simulink model "Overall_Mission"  (R2019b)
settings: Solver=VariableStepAuto  StartTime=0.0  StopTime=10.0  RelTol=1e-3
settings Model: Creator=visha  LastModifiedBy=visha
settings OptimizationCC: DefaultParameterBehavior=Inlined

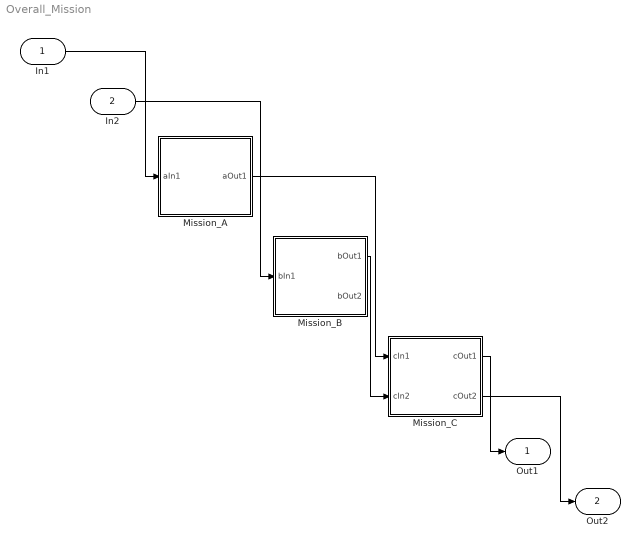
== system Overall_Mission ==
  In1 : Inport  OutDataTypeStr=double
  In2 : Inport  Port=2  OutDataTypeStr=int32
  Mission_A : Subsystem
  Mission_B : Subsystem
  Mission_C : Subsystem
  Out1 : Outport  OutDataTypeStr=double
  Out2 : Outport  Port=2  OutDataTypeStr=boolean
  wires:
  In1/1 -> Mission_A/1(aIn1)
  In2/1 -> Mission_B/1(bIn1)
  Mission_A/1(aOut1) -> Mission_C/1(cIn1)
  Mission_B/1(bOut1) -> Mission_C/2(cIn2)
  Mission_C/1(cOut1) -> Out1/1
  Mission_C/2(cOut2) -> Out2/1

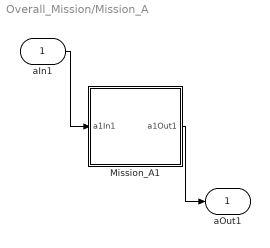
== system Overall_Mission/Mission_A ==
  aIn1 : Inport  OutDataTypeStr=double
  Mission_A1 : Subsystem
  aOut1 : Outport  OutDataTypeStr=double
  wires:
  Mission_A1/1(a1Out1) -> aOut1/1
  aIn1/1 -> Mission_A1/1(a1In1)

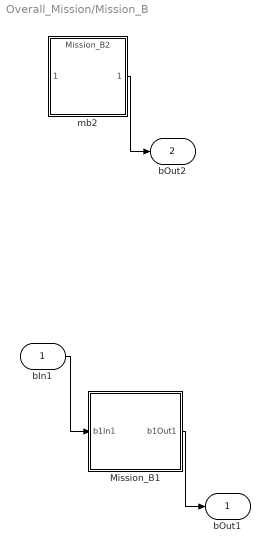
== system Overall_Mission/Mission_B ==
  bIn1 : Inport  OutDataTypeStr=int32
  Mission_B1 : Subsystem
  mb2 : ModelReference  ModelNameDialog=Mission_B2  SimulationMode=Normal  ModelReferenceVersion=1.1
  bOut1 : Outport  OutDataTypeStr=int32
  bOut2 : Outport  Port=2  OutDataTypeStr=int32
  wires:
  bIn1/1 -> Mission_B1/1(b1In1)
  Mission_B1/1(b1Out1) -> bOut1/1
  mb2/1 -> bOut2/1

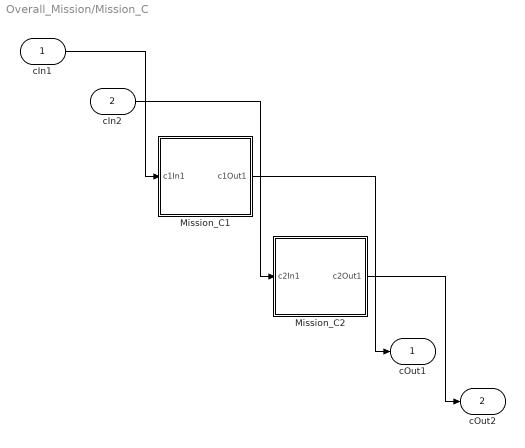
== system Overall_Mission/Mission_C ==
  cIn1 : Inport  OutDataTypeStr=double
  cIn2 : Inport  Port=2  OutDataTypeStr=int32
  Mission_C1 : Subsystem
  Mission_C2 : Subsystem
  cOut1 : Outport  OutDataTypeStr=double
  cOut2 : Outport  Port=2  OutDataTypeStr=boolean
  wires:
  cIn1/1 -> Mission_C1/1(c1In1)
  cIn2/1 -> Mission_C2/1(c2In1)
  Mission_C1/1(c1Out1) -> cOut1/1
  Mission_C2/1(c2Out1) -> cOut2/1

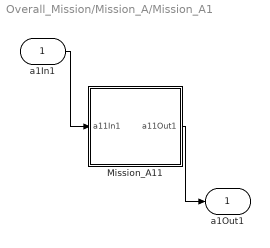
== system Overall_Mission/Mission_A/Mission_A1 ==
  a1In1 : Inport  OutDataTypeStr=double
  Mission_A11 : Subsystem
  a1Out1 : Outport  OutDataTypeStr=double
  wires:
  a1In1/1 -> Mission_A11/1(a11In1)
  Mission_A11/1(a11Out1) -> a1Out1/1

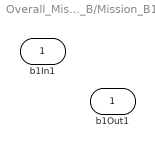
== system Overall_Mission/Mission_B/Mission_B1 ==
  b1In1 : Inport  OutDataTypeStr=int32
  b1Out1 : Outport  OutDataTypeStr=int32

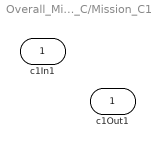
== system Overall_Mission/Mission_C/Mission_C1 ==
  c1In1 : Inport  OutDataTypeStr=double
  c1Out1 : Outport  OutDataTypeStr=double

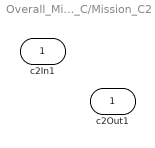
== system Overall_Mission/Mission_C/Mission_C2 ==
  c2In1 : Inport  OutDataTypeStr=int32
  c2Out1 : Outport  OutDataTypeStr=boolean

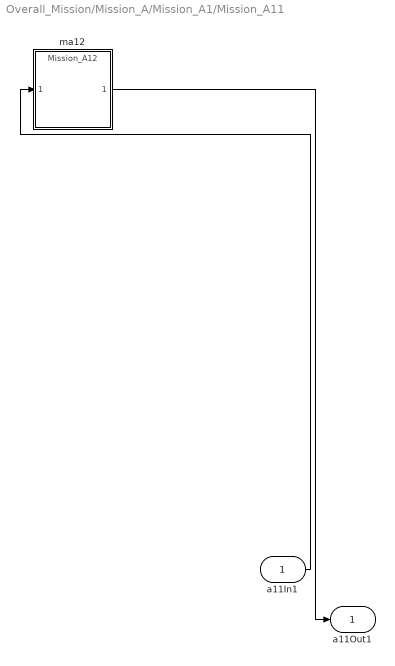
== system Overall_Mission/Mission_A/Mission_A1/Mission_A11 ==
  a11In1 : Inport  OutDataTypeStr=double
  ma12 : ModelReference  ModelNameDialog=Mission_A12  SimulationMode=Normal  ModelReferenceVersion=1.1
  a11Out1 : Outport  OutDataTypeStr=double
  wires:
  a11In1/1 -> ma12/1
  ma12/1 -> a11Out1/1
